simulink model "verify_Pump_Additional_mdl"  (R2016b)
settings: Solver=ode45  StartTime=0.0  StopTime=75  MaxStep=1  RelTol=1e-3  EnableMultiTasking=on
undefined symbols (not defined in the file or in its folder): path_carnot
libraries: carnot x2, simulink x1
settings Model: Creator=drhf  LastModifiedBy=drhf
settings DataIOCC: SaveFormat=Array  SignalLoggingSaveFormat=ModelDataLogs
settings OptimizationCC: ExpressionDepthLimit=2147483647  LifeSpan=inf
settings DebuggingCC: UnderspecifiedInitializationDetection=Classic  MergeDetectMultiDrivingBlocksExec=none  SolverPrmCheckMsg=warning  FcnCallInpInsideContextMsg=warning  StateNameClashWarn=warning  SFUnexpectedBacktrackingDiag=warning  SFNoUnconditionalDefaultTransitionDiag=warning  SFExecutionAtInitializationDiag=none
settings HardwareCC: ProdBitPerPointer=32  ProdBitPerSizeT=32  ProdBitPerPtrDiffT=32  ProdLargestAtomicFloat=None  ProdIntDivRoundTo=Undefined  ProdEndianess=Unspecified  ProdWordSize=32  ProdHWDeviceType=32-bit Generic
settings ModelReferenceCC: PropagateSignalLabelsOutOfModel=off
settings GRTTargetCC: TargetLangStandard=C89/C90 (ANSI)  GeneratePreprocessorConditionals=Disable all  CombineOutputUpdateFcns=off  GRTInterface=on
settings ConfigComp: CovMetricSettings=dw  CovHtmlReporting=on  CovSaveCumulativeToWorkspaceVar=on  CovSaveSingleToWorkspaceVar=on  CovExternalEMLEnable=off

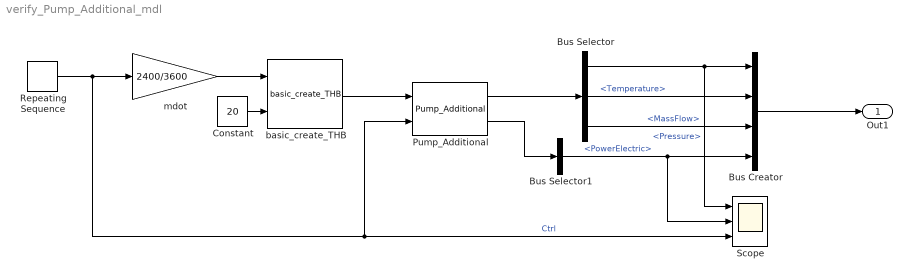
== system verify_Pump_Additional_mdl ==
  Bus Creator : BusCreator  Inputs=4
  Bus Selector : BusSelector  OutputSignals=Pressure,Temperature,MassFlow
  Bus Selector1 : BusSelector  OutputSignals=PowerElectric
  Constant : Constant  Value=20
  Pump_Additional : carnot/Hydraulics/Pump_Additional  Tini=20  PathName=fullfile(path_carnot('libsl'), 'Hydraulics', 'Pump_Main', 'parameter_set')  FileName='Pump5m.mat'  userPath=off  userParam=off  a0=50000  a1=-45000  a2=0  dia=0.02  UA=1  mcp=4182  e0=35  e1=22.5  e2=-8.1
  Repeating Sequence : simulink/Sources/Repeating Sequence  rep_seq_t=[0 20 60 80]  rep_seq_y=[0 0 1 1]
  Scope : Scope  NumInputPorts=3
  basic_create_THB : carnot/Basic/Hydraulics/basic_create_THB  p=2e5  fluid=Water  mix=0  mix2=0  mix3=0  dia=0.02  hgt=0  mID=No Pressure Drop
  mdot : Gain  Gain=2400/3600
  Out1 : Outport
  wires:
  Bus Creator/1 -> Out1/1
  Bus Selector/3 -> Bus Creator/3  "<MassFlow>"
  Repeating Sequence/1 -> mdot/1, Pump_Additional/2, Scope/3  "Ctrl"
  basic_create_THB/1 -> Pump_Additional/1
  Pump_Additional/1 -> Bus Selector/1
  Pump_Additional/2 -> Bus Selector1/1
  Bus Selector/1 -> Scope/1, Bus Creator/1  "<Pressure>"
  Bus Selector/2 -> Bus Creator/2  "<Temperature>"
  Bus Selector1/1 -> Scope/2, Bus Creator/4  "<PowerElectric>"
  Constant/1 -> basic_create_THB/2
  mdot/1 -> basic_create_THB/1
